simulink model "untitled"  (R2017b)
settings: Solver=FixedStepAuto  StartTime=0.0  StopTime=0.08  FixedStep=5e-6  RelTol=1e-3
undefined symbols (not defined in the file): fdesignblkfcn, gcbh
libraries: simulink x1, dspfdesign x1, dsparch4 x1, powerlib x1
(part 3 of 3)

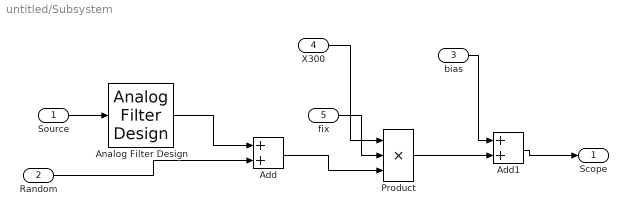
== system untitled/Subsystem ==
  Source : Inport
  Random : Inport  Port=2
  bias : Inport  Port=3
  X300 : Inport  Port=4
  fix : Inport  Port=5
  Add : Sum
  Add1 : Sum
  Analog Filter Design : dsparch4/Analog Filter Design  method=Butterworth  filttype=Lowpass  N=5  Wlo=400*2*pi  Whi=80  Rp=2  Rs=40
  Product : Product  Inputs=3
  Scope : Outport
  wires:
  Analog Filter Design/1 -> Add/1
  Source/1 -> Analog Filter Design/1
  Random/1 -> Add/2
  bias/1 -> Add1/1
  Add1/1 -> Scope/1
  Product/1 -> Add1/2
  Add/1 -> Product/3
  fix/1 -> Product/2
  X300/1 -> Product/1

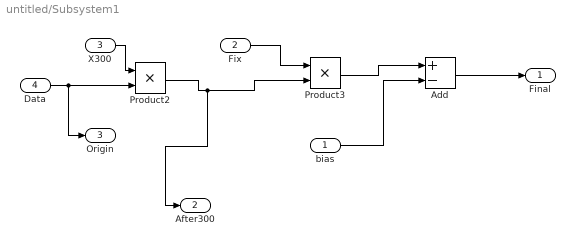
== system untitled/Subsystem1 ==
  bias : Inport
  Fix : Inport  Port=2
  X300 : Inport  Port=3
  Data : Inport  Port=4
  Add : Sum  Inputs=+-
  Product2 : Product
  Product3 : Product
  Final : Outport
  After300 : Outport  Port=2
  Origin : Outport  Port=3
  wires:
  X300/1 -> Product2/1
  Fix/1 -> Product3/1
  Product2/1 -> After300/1, Product3/2
  Data/1 -> Origin/1, Product2/2
  Add/1 -> Final/1
  Product3/1 -> Add/1
  bias/1 -> Add/2

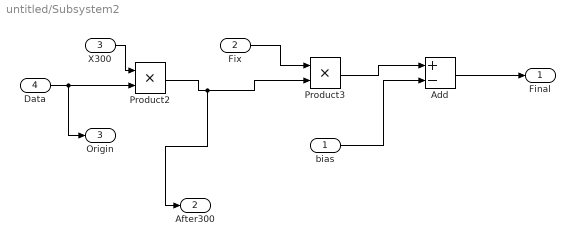
== system untitled/Subsystem2 ==
  bias : Inport
  Fix : Inport  Port=2
  X300 : Inport  Port=3
  Data : Inport  Port=4
  Add : Sum  Inputs=+-
  Product2 : Product
  Product3 : Product
  Final : Outport
  After300 : Outport  Port=2
  Origin : Outport  Port=3
  wires:
  X300/1 -> Product2/1
  Fix/1 -> Product3/1
  Product2/1 -> After300/1, Product3/2
  Data/1 -> Origin/1, Product2/2
  Add/1 -> Final/1
  Product3/1 -> Add/1
  bias/1 -> Add/2

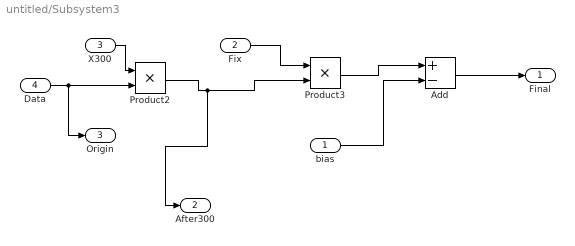
== system untitled/Subsystem3 ==
  bias : Inport
  Fix : Inport  Port=2
  X300 : Inport  Port=3
  Data : Inport  Port=4
  Add : Sum  Inputs=+-
  Product2 : Product
  Product3 : Product
  Final : Outport
  After300 : Outport  Port=2
  Origin : Outport  Port=3
  wires:
  X300/1 -> Product2/1
  Fix/1 -> Product3/1
  Product2/1 -> After300/1, Product3/2
  Data/1 -> Origin/1, Product2/2
  Add/1 -> Final/1
  Product3/1 -> Add/1
  bias/1 -> Add/2

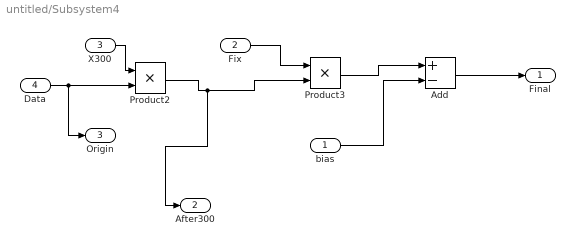
== system untitled/Subsystem4 ==
  bias : Inport
  Fix : Inport  Port=2
  X300 : Inport  Port=3
  Data : Inport  Port=4
  Add : Sum  Inputs=+-
  Product2 : Product
  Product3 : Product
  Final : Outport
  After300 : Outport  Port=2
  Origin : Outport  Port=3
  wires:
  X300/1 -> Product2/1
  Fix/1 -> Product3/1
  Product2/1 -> After300/1, Product3/2
  Data/1 -> Origin/1, Product2/2
  Add/1 -> Final/1
  Product3/1 -> Add/1
  bias/1 -> Add/2

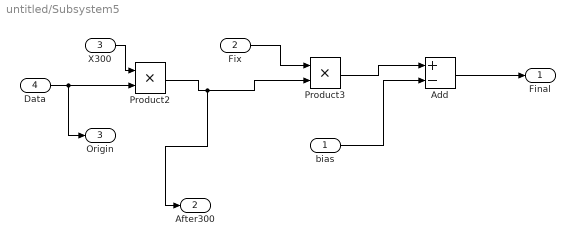
== system untitled/Subsystem5 ==
  bias : Inport
  Fix : Inport  Port=2
  X300 : Inport  Port=3
  Data : Inport  Port=4
  Add : Sum  Inputs=+-
  Product2 : Product
  Product3 : Product
  Final : Outport
  After300 : Outport  Port=2
  Origin : Outport  Port=3
  wires:
  X300/1 -> Product2/1
  Fix/1 -> Product3/1
  Product2/1 -> After300/1, Product3/2
  Data/1 -> Origin/1, Product2/2
  Add/1 -> Final/1
  Product3/1 -> Add/1
  bias/1 -> Add/2
